simulink model "backstepping_compliant"  (R2022b)
settings: Solver=VariableStepAuto  StartTime=0.0  StopTime=30.0  RelTol=1e-3
undefined symbols (not defined in the file or in its folder): Lamda
settings Model: Creator=alexi  LastModifiedBy=alexi

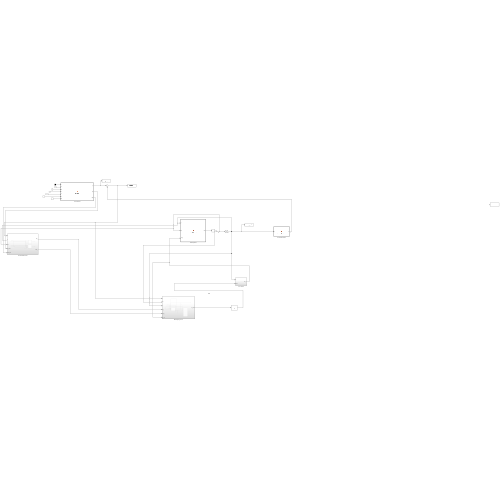
[thumbnail: Simulink's stored preview of the top-level diagram]
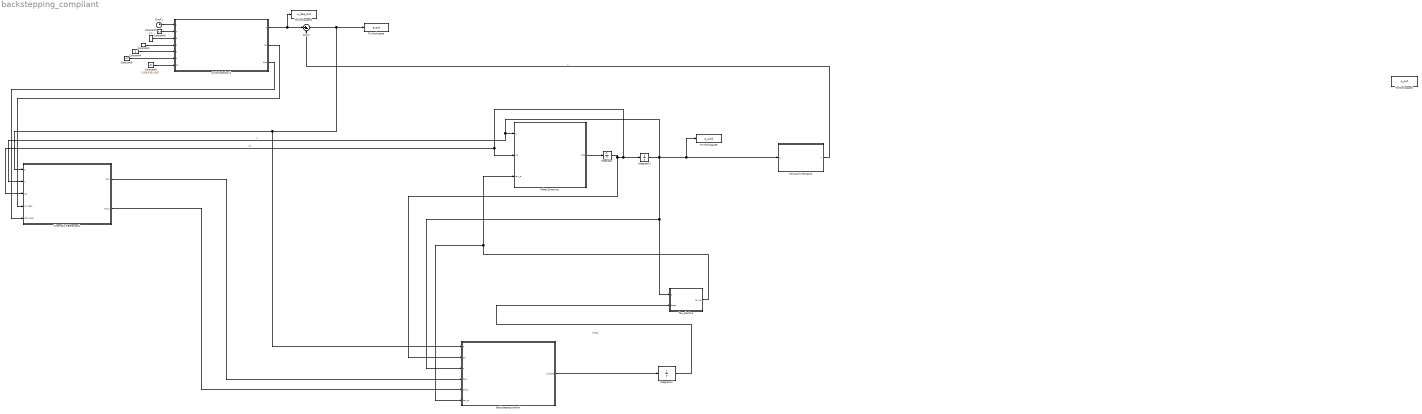
== system backstepping_compliant ==
  note: theta
  Backstepping control : Subsystem
  Clock1 : Clock
  Constant2 : Constant  Value=0.4
  Constant3 : Constant
  Constant4 : Constant  Value=2
  Constant5 : Constant  Value=1.57
  Constant6 : Constant  Value=[0.85,0.85,0.85]
  Constant9 : Constant  Value=0.4
  Forward Kinematics : MATLAB Function  TreatAsAtomicUnit=on
  Integrator : Integrator  InitialCondition=[0,0,0]'
  Integrator1 : Integrator  InitialCondition=[0.25,0.25,0.25]'
  Integrator2 : Integrator  InitialCondition=[0,0,0]
  Kinematic References1 : Subsystem
  Robot Dynamics : MATLAB Function  TreatAsAtomicUnit=on
  Sum4 : Sum  Inputs=|+-
  Tau_elastica : Subsystem
  To Workspace : ToWorkspace  VariableName=e_out  SaveFormat=Timeseries  SampleTime=-1
  To Workspace1 : ToWorkspace  VariableName=xi_des_out  SaveFormat=Timeseries  SampleTime=-1
  To Workspace2 : ToWorkspace  VariableName=q_out  SaveFormat=Timeseries  SampleTime=-1
  To Workspace3 : ToWorkspace  VariableName=q_out1  SaveFormat=Timeseries  SampleTime=-1
  circle trajectory1 : MATLAB Function  TreatAsAtomicUnit=on
  wires:
  Clock1/1 -> circle trajectory1/1(t)
  Constant9/1 -> circle trajectory1/2(A)
  Constant2/1 -> circle trajectory1/3(B)
  Constant3/1 -> circle trajectory1/4(a)
  Constant4/1 -> circle trajectory1/5(b)
  Constant5/1 -> circle trajectory1/6(d)
  Constant6/1 -> circle trajectory1/7(p0)
  Integrator/1 -> Backstepping control/2(dq), Integrator1/1, Robot Dynamics/2(dq), Kinematic References1/3(dq)  "dq"
  Robot Dynamics/1(ddq) -> Integrator/1
  Integrator1/1 -> Tau_elastica/1(q), Backstepping control/3(q), Kinematic References1/2(q), Robot Dynamics/1(q), Forward Kinematics/1(q), To Workspace3/1  "q"
  circle trajectory1/1(p) -> To Workspace1/1, Sum4/1
  Forward Kinematics/1(xi) -> Sum4/2  "xi"
  Sum4/1 -> To Workspace/1, Backstepping control/1(e), Kinematic References1/1(e)
  circle trajectory1/2(dp) -> Kinematic References1/4(dxi_des)
  circle trajectory1/3(ddp) -> Kinematic References1/5(ddxi_des)
  Tau_elastica/1(tau_el) -> Robot Dynamics/3(tau_el), Backstepping control/6(tau_el)
  Integrator2/1 -> Tau_elastica/2(theta)
  Kinematic References1/1(dq_r) -> Backstepping control/4(dq_r)
  Kinematic References1/2(ddq_r) -> Backstepping control/5(ddq_r)
  Backstepping control/1(d_theta) -> Integrator2/1

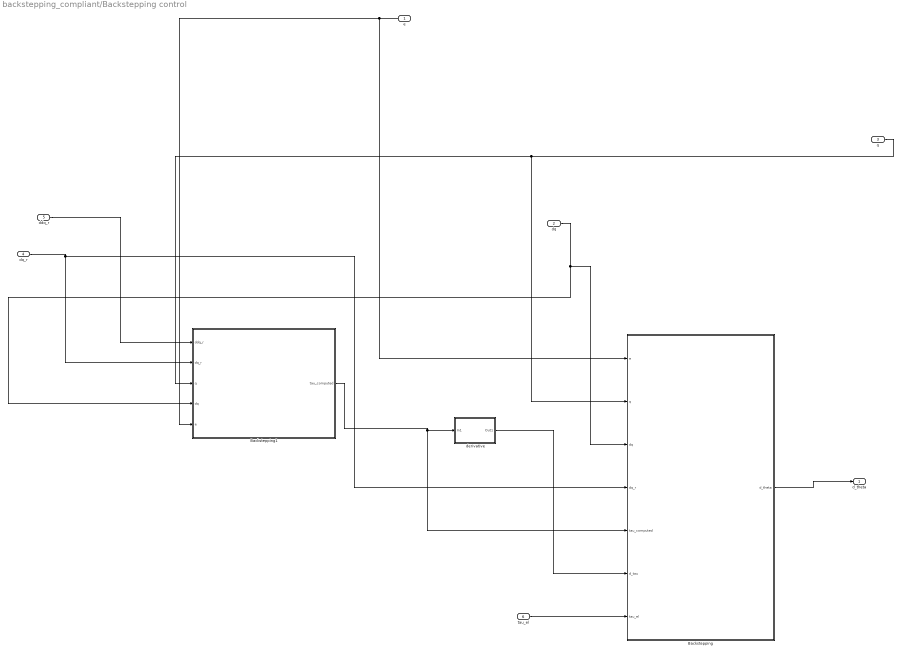
== system backstepping_compliant/Backstepping control ==
  e : Inport
  dq : Inport  Port=2
  q : Inport  Port=3
  dq_r : Inport  Port=4
  ddq_r : Inport  Port=5
  tau_el : Inport  Port=6
  Backstepping : MATLAB Function  TreatAsAtomicUnit=on
  Backstepping1 : MATLAB Function  TreatAsAtomicUnit=on
  derivative : Subsystem
  d_theta : Outport
  wires:
  dq_r/1 -> Backstepping/4(dq_r), Backstepping1/2(dq_r)
  derivative/1(Out1) -> Backstepping/6(d_tau)
  q/1 -> Backstepping/2(q), Backstepping1/3(q)
  Backstepping1/1(tau_computed) -> Backstepping/5(tau_computed), derivative/1(In1)
  e/1 -> Backstepping/1(e), Backstepping1/5(e)
  tau_el/1 -> Backstepping/7(tau_el)
  ddq_r/1 -> Backstepping1/1(ddq_r)
  dq/1 -> Backstepping1/4(dq), Backstepping/3(dq)
  Backstepping/1(d_theta) -> d_theta/1

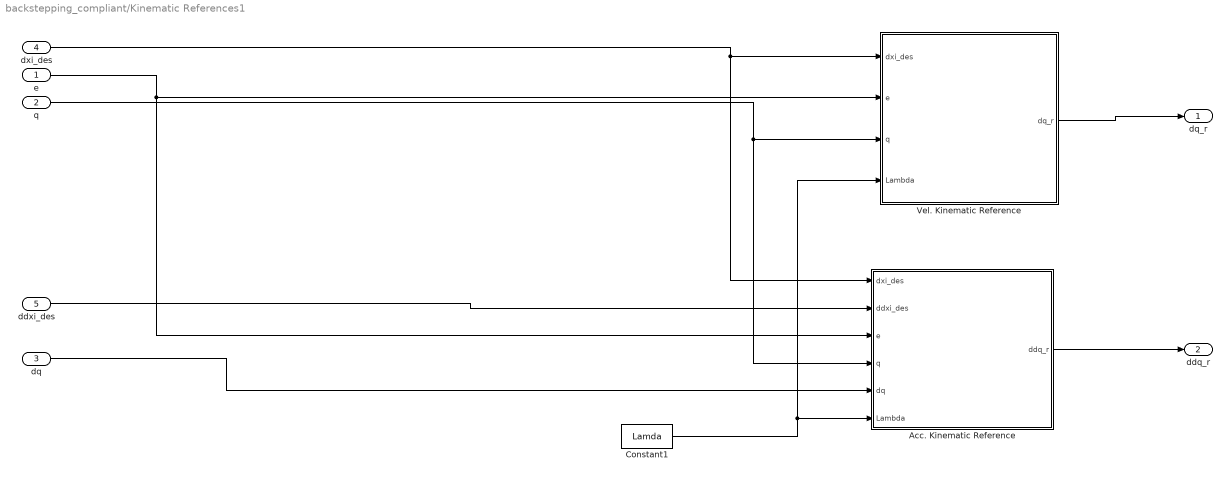
== system backstepping_compliant/Kinematic References1 ==
  e : Inport
  q : Inport  Port=2
  dq : Inport  Port=3
  dxi_des : Inport  Port=4
  ddxi_des : Inport  Port=5
  Acc. Kinematic Reference : MATLAB Function  TreatAsAtomicUnit=on
  Constant1 : Constant  Value=Lamda
  "Vel. Kinematic Reference " : MATLAB Function  TreatAsAtomicUnit=on
  dq_r : Outport  VectorParamsAs1DForOutWhenUnconnected=off
  ddq_r : Outport  Port=2  VectorParamsAs1DForOutWhenUnconnected=off
  wires:
  ddxi_des/1 -> Acc. Kinematic Reference/2(ddxi_des)
  e/1 -> Acc. Kinematic Reference/3(e), "Vel. Kinematic Reference "/2(e)
  dxi_des/1 -> Acc. Kinematic Reference/1(dxi_des), "Vel. Kinematic Reference "/1(dxi_des)
  Constant1/1 -> "Vel. Kinematic Reference "/4(Lambda), Acc. Kinematic Reference/6(Lambda)
  "Vel. Kinematic Reference "/1(dq_r) -> dq_r/1
  dq/1 -> Acc. Kinematic Reference/5(dq)
  q/1 -> Acc. Kinematic Reference/4(q), "Vel. Kinematic Reference "/3(q)
  Acc. Kinematic Reference/1(ddq_r) -> ddq_r/1

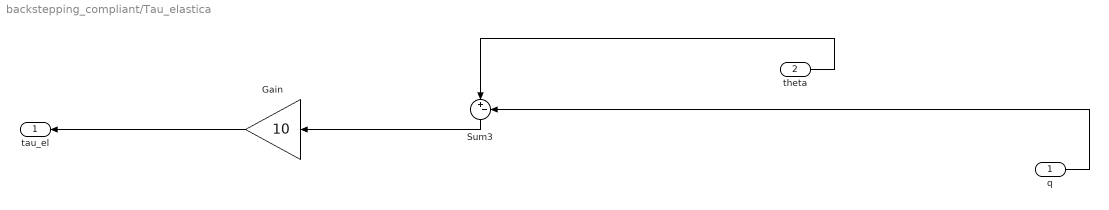
== system backstepping_compliant/Tau_elastica ==
  q : Inport
  theta : Inport  Port=2
  Gain : Gain  Gain=10
  Sum3 : Sum  Inputs=|+-
  tau_el : Outport
  wires:
  Sum3/1 -> Gain/1
  q/1 -> Sum3/2
  Gain/1 -> tau_el/1
  theta/1 -> Sum3/1

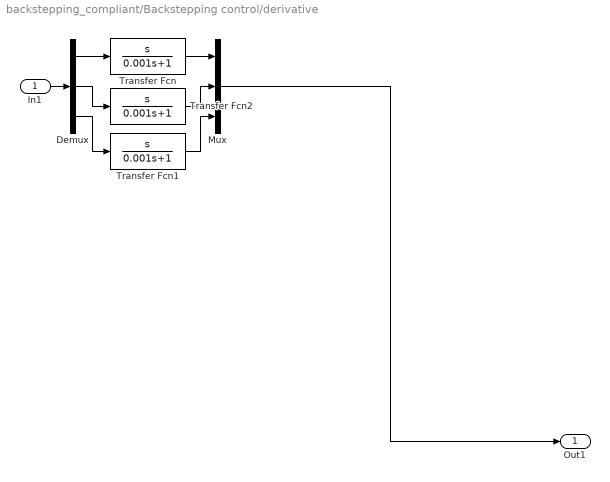
== system backstepping_compliant/Backstepping control/derivative ==
  In1 : Inport
  Demux : Demux  Outputs=3
  Mux : Mux  Inputs=3
  Transfer Fcn : TransferFcn  Numerator=[1 0]  Denominator=[0.001 1]
  Transfer Fcn1 : TransferFcn  Numerator=[1 0]  Denominator=[0.001 1]
  Transfer Fcn2 : TransferFcn  Numerator=[1 0]  Denominator=[0.001 1]
  Out1 : Outport
  wires:
  Transfer Fcn1/1 -> Mux/3
  Demux/3 -> Transfer Fcn1/1
  In1/1 -> Demux/1
  Mux/1 -> Out1/1
  Demux/2 -> Transfer Fcn2/1
  Transfer Fcn2/1 -> Mux/2
  Transfer Fcn/1 -> Mux/1
  Demux/1 -> Transfer Fcn/1

== matlab function backstepping_compliant/Backstepping control/Backstepping1 ==
  data: ddq_r input; dq_r input; q input; dq input; e input; tau_computed output
function tau_computed  = computed_torque(ddq_r,dq_r,q,dq,e)

coder.extrinsic('disp');
rel_err = 0;
de = dq_r-dq;
Kp = 100;
Kv = 100;
% Get dynamic matrices
B = RRR_mass_matrix(q);
C = RRR_coriolis_matrix(q,dq);
G = RRR_gravity_matrix(q);

% Adding uncertainty
B = B.*(1 + rel_err);
C = C.*(1 + rel_err);
G = G.*(1 + rel_err);

a1 = 1;
a2 = 1;
a3 = 1;
q1 = q(1);
q2 = q(2);
q3 = q(3);
% Get Jacobian
% J = [- a1*sin(q1) - a3*cos(q3)*(sin(q1+q2)) - a2*sin(q1+q2), -a3*cos(q3)*(sin(q1+q2)) - a2*sin(q1+q2), -a3*sin(q3)*(cos(q1+q2)); ...
%     a1*cos(q1) + a3*cos(q3)*(cos(q1+q2)) + a2*cos(q1+q2),   a3*cos(q3)*(cos(q1+q2)) + a2*cos(q1+q2),  -a3*sin(q3)*(sin(q1+q2)); ...
%     0,0,- a3*cos(q3)*(sin(q1+q2))^2 - a3*cos(q3)*(cos(q1+q2))^2];

% Control law
tau_computed = B*ddq_r+C*dq+G+B*Kp*e+B*Kv*de;

== matlab function backstepping_compliant/circle trajectory1 ==
  data: t input; p output; dp output; ddp output; A input; B input; a input; b input; d input; p0 input
function [p,dp,ddp] = lissajous(t,A,B,a,b,d,p0)
C = 0.1;  % Ampiezza dell'oscillazione in z
c = 0.2;  % Frequenza in z
phi = pi/4;
p = [A*sin(a*t+d); B*sin(b*t);C*sin(c*t + phi)] + p0;
dp = [A*a*cos(a*t+d); B*b*cos(b*t);C*c*cos(c*t+phi)];
ddp = [-A*a^2*sin(a*t+d); -B*b^2*sin(b*t);-C*c^2*sin(c*t+phi)];
% a = 0.2;    % Ampiezza lungo l'asse X
% b = 0.2;    % Ampiezza lungo l'asse Y
% p0 = [1;0.8;0.8];
% 
% x = a * cos(t);
% y = b * sin(t);
% z =  0.1 * sin(t);
% 
% p = [x y z]'+p0;
% 
% dx = -a*sin(t);
% dy = b*cos(t);
% dz = 0.5*cos(t);
% 
% dp = [dx dy dz]';
% 
% ddx = -a*cos(t);
% ddy = -b*sin(t);
% ddz = -0.5*sin(t);
% 
% ddp = [ddx ddy ddz]';

== matlab function backstepping_compliant/Backstepping control/Backstepping ==
  data: e input; q input; dq input; dq_r input; tau_computed input; d_tau input; d_theta output; tau_el input
function d_theta  = backstepping(e,q,dq,dq_r,tau_computed,d_tau,tau_el)

coder.extrinsic('disp');
rel_err = 0;
de = dq_r-dq;
P = 30*eye(3);
K = 10;
Kp = 100;

% Get dynamic matrices
B = RRR_mass_matrix(q);
C = RRR_coriolis_matrix(q,dq);
G = RRR_gravity_matrix(q);

% Adding uncertainty
B = B.*(1 + rel_err);
C = C.*(1 + rel_err);
G = G.*(1 + rel_err);
g = [zeros(3,3); -pinv(B)];

a1 = 1;
a2 = 1;
a3 = 1;
q1 = q(1);
q2 = q(2);
q3 = q(3);
% Get Jacobian
% J = [- a1*sin(q1) - a3*cos(q3)*(sin(q1+q2)) - a2*sin(q1+q2), -a3*cos(q3)*(sin(q1+q2)) - a2*sin(q1+q2), -a3*sin(q3)*(cos(q1+q2)); ...
%     a1*cos(q1) + a3*cos(q3)*(cos(q1+q2)) + a2*cos(q1+q2),   a3*cos(q3)*(cos(q1+q2)) + a2*cos(q1+q2),  -a3*sin(q3)*(sin(q1+q2)); ...
%     0,0,- a3*cos(q3)*(sin(q1+q2))^2 - a3*cos(q3)*(cos(q1+q2))^2];

% Control law
%d_theta = B*ddq_r + C*dq_r + G + Ks*de + J.'*e;
Vx1 = [e'*Kp,de'];
l = K;
h = -K*dq;
v = d_tau+pinv(P)*(K*(tau_computed-tau_el)-g'*Vx1');
d_theta = inv(l)*(v-h);

== matlab function backstepping_compliant/Robot Dynamics ==
  data: q input; dq input; tau_el input; ddq output
function ddq = inverse_dynamics(q,dq, tau_el)

% Get dynamic matrices
B = RRR_mass_matrix(q);
C = RRR_coriolis_matrix(q,dq);
G = RRR_gravity_matrix(q);
ddq = pinv(B)*(tau_el - C*dq - G);

== matlab function backstepping_compliant/Forward Kinematics ==
  data: q input; xi output
function xi  = RR_forward_kinematics(q)

    q1 = q(1);
    q2 = q(2);
    q3 = q(3);

    a1 = 1;
    a2 = 1;
    a3 = 1;

    p0 = [0;0;0];
    p1 = [a1*cos(q1); a1*sin(q1);0];
    p2 = p1+[a2*cos(q1+q2);a2*sin(a1+q2);0];
    xi = [a1*cos(q1) + a3*cos(q3)*(cos(q1)*cos(q2) - sin(q1)*sin(q2)) + a2*cos(q1)*cos(q2) - a2*sin(q1)*sin(q2); a1*sin(q1) + a3*cos(q3)*(cos(q1)*sin(q2) + cos(q2)*sin(q1)) + a2*cos(q1)*sin(q2) + a2*cos(q2)*sin(q1);-a3*sin(q3)];
end

== matlab function backstepping_compliant/Kinematic References1/Acc. Kinematic Reference ==
  data: dxi_des input; ddq_r output; ddxi_des input; e input; q input; dq input; Lambda input
function ddq_r = acc_kinematic_reference(dxi_des, ddxi_des, e, q, dq, Lambda)

coder.extrinsic('disp');

J = zeros(3,3);
dJ = zeros(3,3);

dq1 = dq(1);
dq2 = dq(2);
dq3 = dq(3);

q1 = q(1);
q2 = q(2);
q3 = q(3);

a1 = 1;
a2 = 1;
a3 = 1;

% Computing jacobian and derivative
J = [- a1*sin(q1) - a3*cos(q3)*(cos(q1)*sin(q2) + cos(q2)*sin(q1)) - a2*cos(q1)*sin(q2) - a2*cos(q2)*sin(q1), -a3*cos(q3)*(cos(q1)*sin(q2) +cos(q2)*sin(q1)) - a2*cos(q1)*sin(q2) - a2*cos(q2)*sin(q1), -a3*sin(q3)*(cos(q1)*cos(q2) - sin(q1)*sin(q2)); ...
    a1*cos(q1) + a3*cos(q3)*(cos(q1)*cos(q2) - sin(q1)*sin(q2)) + a2*cos(q1)*cos(q2) - a2*sin(q1)*sin(q2),   a3*cos(q3)*(cos(q1)*cos(q2) - sin(q1)*sin(q2)) + a2*cos(q1)*cos(q2) - a2*sin(q1)*sin(q2),  -a3*sin(q3)*(cos(q1)*sin(q2) + cos(q2)*sin(q1)); ...
    0,0,- a3*cos(q3)*(cos(q1)*sin(q2) + cos(q2)*sin(q1))^2 - a3*cos(q3)*(cos(q1)*cos(q2) - sin(q1)*sin(q2))^2];

a11 = -a1*dq1*cos(q1)-a3*(dq1*cos(q1+q2)+ dq2*cos(q1+q2))*sin(q3)-a2*(dq1*cos(q1+q2)+ dq2*cos(q1+q2));
a12 = -a3*( dq1*cos(q1+q2)+ dq2*cos(q1+q2))*sin(q3)-a2*( dq1*cos(q1+q2)+ dq2*cos(q1+q2));
a13 = -a3*( dq1*cos(q1+q2)+ dq2*cos(q1+q2))*cos(q3);
a21 = -a1*dq1*sin(q1)-a3*( dq1*sin(q1+q2)+ dq2*sin(q1+q2))*cos(q3)-a2*( dq1*sin(q1+q2)+ dq2*sin(q1+q2));
a22 = -a3*(dq1*sin(q1+q2)+dq2*sin(q1+q2))*sin(q3)-a2*(dq1*sin(q1+q2)+dq2*sin(q1+q2));
a23 = -a3*(dq1*cos(q1+q2)+dq2*cos(q1+q2))*sin(q3);
a31 = 0;
a32 = 0;
a33 = 2*a3*(dq1*cos(q1+q2)+dq2*cos(q1+q2))*sin(q1+q2)*sin(q3)-2*a3*(dq1*sin(q1+q2)+dq2*sin(q1+q2))*cos(q1+q2)*sin(q3);

dJ = [a11,a12,a13;a21,a22,a23;a31,a32,a33];

ddq_r = inv(J) * (ddxi_des + Lambda*dxi_des - Lambda*J*dq) ...
- inv(J)*dJ*inv(J)*(dxi_des + Lambda*e);
end

== matlab function backstepping_compliant/Kinematic References1/Vel. Kinematic Reference  ==
  data: dxi_des input; dq_r output; e input; q input; Lambda input
function dq_r = vel_kinematic_reference(dxi_des, e, q, Lambda)
a1 = 1;
a2 = 1;
a3 = 1;

q1 = q(1);
q2 = q(2);
q3 = q(3);

% Computing jacobian
J = [- a1*sin(q1) - a3*cos(q3)*(cos(q1)*sin(q2) + cos(q2)*sin(q1)) - a2*cos(q1)*sin(q2) - a2*cos(q2)*sin(q1), -a3*cos(q3)*(cos(q1)*sin(q2) +cos(q2)*sin(q1)) - a2*cos(q1)*sin(q2) - a2*cos(q2)*sin(q1), -a3*sin(q3)*(cos(q1)*cos(q2) - sin(q1)*sin(q2)); ...
    a1*cos(q1) + a3*cos(q3)*(cos(q1)*cos(q2) - sin(q1)*sin(q2)) + a2*cos(q1)*cos(q2) - a2*sin(q1)*sin(q2),   a3*cos(q3)*(cos(q1)*cos(q2) - sin(q1)*sin(q2)) + a2*cos(q1)*cos(q2) - a2*sin(q1)*sin(q2),  -a3*sin(q3)*(cos(q1)*sin(q2) + cos(q2)*sin(q1)); ...
    0,0,- a3*cos(q3)*(cos(q1)*sin(q2) + cos(q2)*sin(q1))^2 - a3*cos(q3)*(cos(q1)*cos(q2) - sin(q1)*sin(q2))^2];

dq_r = inv(J) * (dxi_des + Lambda*e);
end
